simulink model "cascatinha__true_gab"  (R2023a)
settings: Solver=VariableStepAuto  StartTime=0.0  StopTime=7  RelTol=1e-3
values from neighbouring files (symbols this model uses):
  G_roll_thetap = minreal(G_roll_v1/G_thetap_v1)    [Modelo_mono.m]
  G_thetap_v1 = minreal(G(3,1))    [Modelo_mono.m]
undefined symbols (not defined in the file or in its folder): C1_roll, C2_roll
settings Model: Creator=gabri  LastModifiedBy=pinki
settings OptimizationCC: ReuseModelBlockBuffer=off

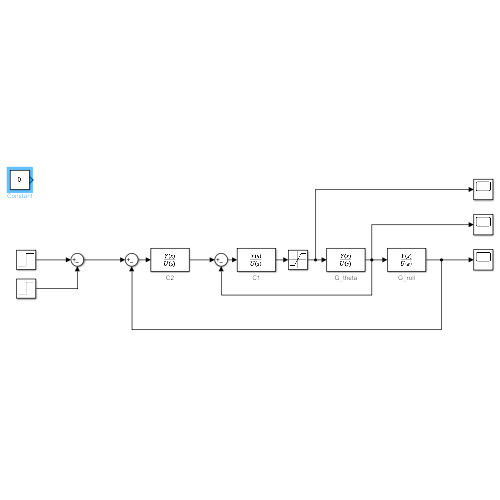
[thumbnail: Simulink's stored preview of the top-level diagram]
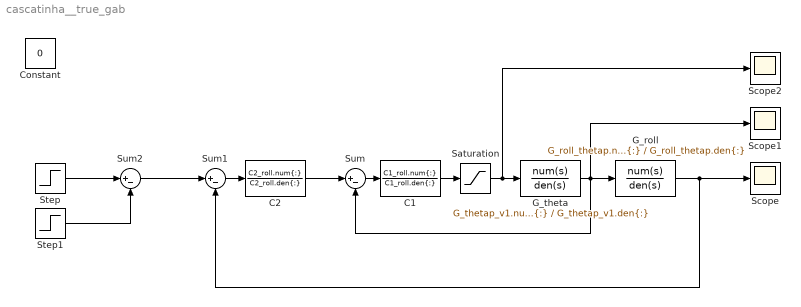
== system cascatinha__true_gab ==
  C1 : TransferFcn  Numerator=C1_roll.num{:}  Denominator=C1_roll.den{:}
  C2 : TransferFcn  Numerator=C2_roll.num{:}  Denominator=C2_roll.den{:}
  Constant : Constant  Value=0
  G_roll : TransferFcn  Numerator=G_roll_thetap.num{:}  Denominator=G_roll_thetap.den{:}
  G_theta : TransferFcn  Numerator=G_thetap_v1.num{:}  Denominator=G_thetap_v1.den{:}
  Saturation : Saturate  UpperLimit=12  LowerLimit=-12
  Scope : Scope
  Scope1 : Scope
  Scope2 : Scope
  Step : Step  After=0.1  SampleTime=0
  Step1 : Step  Time=1.2  After=0.1  SampleTime=0
  Sum : Sum  Inputs=|+-
  Sum1 : Sum  Inputs=|+-
  Sum2 : Sum  Inputs=|+-
  wires:
  C1/1 -> Saturation/1
  Sum/1 -> C1/1
  G_roll/1 -> Scope/1, Sum1/2
  Sum1/1 -> C2/1
  C2/1 -> Sum/1
  G_theta/1 -> Scope1/1, G_roll/1, Sum/2
  Sum2/1 -> Sum1/1
  Step/1 -> Sum2/1
  Step1/1 -> Sum2/2
  Saturation/1 -> Scope2/1, G_theta/1
